simulink model "ThisOne-merged"  (R2026a)
settings: Solver=ode3  StopTime=2  FixedStep=1e-6  EnableMultiTasking=on
PreLoadFcn:
  | BLDCSpeedControlData;
values from neighbouring files (symbols this model uses):
  Jm = 4.97    [BLDCSpeedControlDataNewParam.m]
  p = 4    [BLDCSpeedControlDataNewParam.m]
undefined symbols (not defined in the file or in its folder): Ct_CqToRPM, Down, Up
libraries: nesl_utility x13, fl_lib x9, ee_lib x5, eeGeneralControl x2, eeBldcCurrentController x1, batt_lib x1, slpidlib x1, SignalEditorBlockLib x1
(part 1 of 2)
CloseFcn:
  | try,close(h1_BLDCSpeedControl),end
  | clear h1_BLDCSpeedControl
  | 
  | clear simlog_BLDCSpeedControl
  | clear logsout_BLDCSpeedControl
Description:
  | BLDC Speed Control
settings Model: PauseTimes=0.45  NumberOfSteps=10  Creator=The MathWorks, Inc.
settings DataIOCC: MaxDataPoints=210000  SignalLoggingName=logsout_BLDCSpeedControl
settings SimscapeCC: SimscapeNormalizeSystem=off  SimscapeNominalValues="[{\"value\":\"1\",\"unit\":\"A\"},{\"value\":\"1\",\"unit\":\"bar\"},{\"value\":\"1\",\"unit\":\"cm^2\"},{\"value\":\"1\",\"unit\":\"cm^3/s\"},{\"value\":\"1\",\"unit\":\"kJ/kg\"},{\"value\":\"1\",\"unit\":\"kW\"},{\"value\":\"1\",\"unit\":\"l\"},{\"value\":\"1\",\"unit\":\"N\"},{\"value\":\"1\",\"unit\":\"N*m\"},{\"value\":\"1\",\"unit\":\"V\"}]"  SimscapeLogSimulationStatistics=on  SimscapeLogName=simlog_BLDCSpeedControl  SimscapeLogLimitData=off  SimscapeLogDataHistory=210000.0

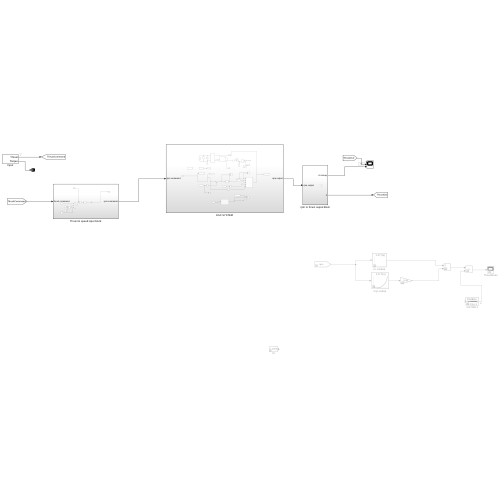
[thumbnail: Simulink's stored preview of the top-level diagram]
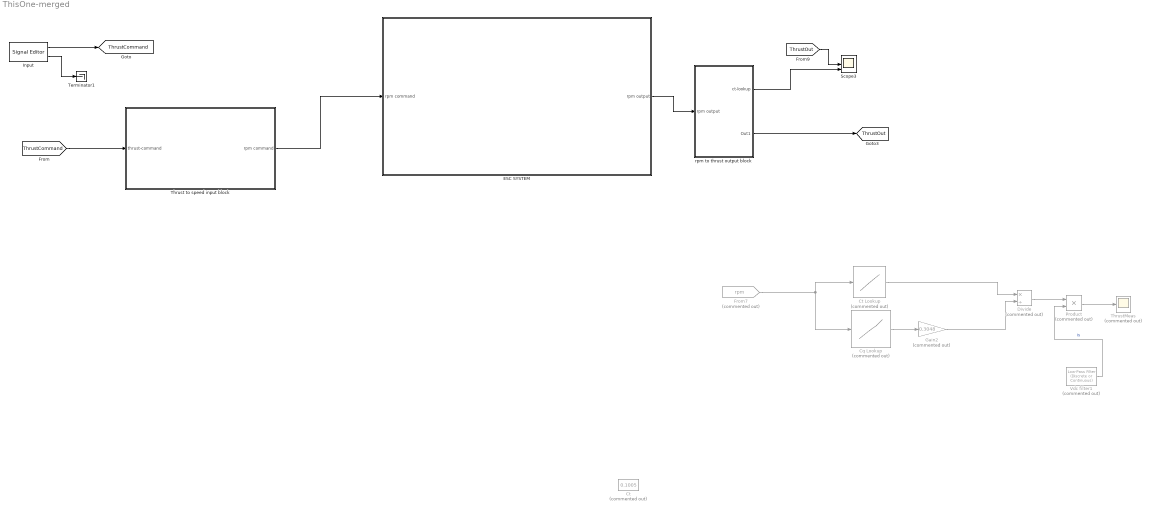
== system ThisOne-merged ==
  Cq Lookup : Lookup_n-D  Commented=on  NumberOfTableDimensions=1  BreakpointsForDimension1=Ct_CqToRPM.RPM  Table=Ct_CqToRPM.Cq  InternalRulePriority=Speed  RndMeth=Simplest
  Ct : Constant  Commented=on  Value=0.1005
  Ct Lookup : Lookup_n-D  Commented=on  NumberOfTableDimensions=1  BreakpointsForDimension1=Ct_CqToRPM.RPM  Table=Ct_CqToRPM.Ct  InternalRulePriority=Speed  RndMeth=Simplest
  Divide : Product  Commented=on  Inputs=*/
  ESC SYSTEM : Subsystem
  From7 : From  Commented=on  GotoTag=rpm  TagVisibility=global
  Gain2 : Gain  Commented=on  Gain=0.3048
  Input : SignalEditorBlockLib/Signal Editor  FileName=BLDCSpeedControlInput.mat  ActiveScenario=Test_1  ActiveSignal=Torque  IsBus=off  OutputBusObjectStr=Bus: BusObject  SampleTime=0  OutputAfterFinalValue=Extrapolation  Unit=inherit  PreserveSignalName=on  ApplySigPropsToAllScenarios=on  ApplySigPropsToAllSignals=off  SignalPropertySource=Dialog parameters
  Product : Product  Commented=on
  Scope3 : Scope  NumInputPorts=3
      settings: ActiveDisplayYMinimum=6.4992210204296432  ActiveDisplayYMaximum=7.577007831129519  DataLoggingVariableName=ScopeData11
  Terminator1 : Terminator
  Thrust to speed input block : Subsystem
  ThrustMeas : Scope  Commented=on
      settings: ActiveDisplayYMinimum=-0.61696410930468792  ActiveDisplayYMaximum=-0.5584126706390744  DataLoggingVariableName=ScopeData2
  Vdc filter1 : eeGeneralControl/Low-Pass Filter (Discrete or Continuous)  Commented=on  K=1  T=0.01  B=inf  A=-inf  init_option=Inherited from block input  x0=0  Ts=-1
  rpm to thrust output block : Subsystem
  tag scope: ThrustCommand=global, ThrustOut=global
  wires:
  Input/2 -> Terminator1/1
  Divide/1 -> Product/1
  Product/1 -> ThrustMeas/1
  Vdc filter1/1 -> Product/2  "is"
  From7/1 -> Cq Lookup/1, Ct Lookup/1
  Ct Lookup/1 -> Divide/1
  Gain2/1 -> Divide/2
  Cq Lookup/1 -> Gain2/1
  [ThrustOut] -> Scope3/2
  Thrust to speed input block/1(rpm command) -> ESC SYSTEM/1(rpm command)
  rpm to thrust output block/1(ct-lookup) -> Scope3/3
  rpm to thrust output block/2(Out1) -> [ThrustOut]
  Input/1 -> [ThrustCommand]
  [ThrustCommand] -> Thrust to speed input block/1(thrust-command)
  ESC SYSTEM/1(rpm output) -> rpm to thrust output block/1(rpm output)

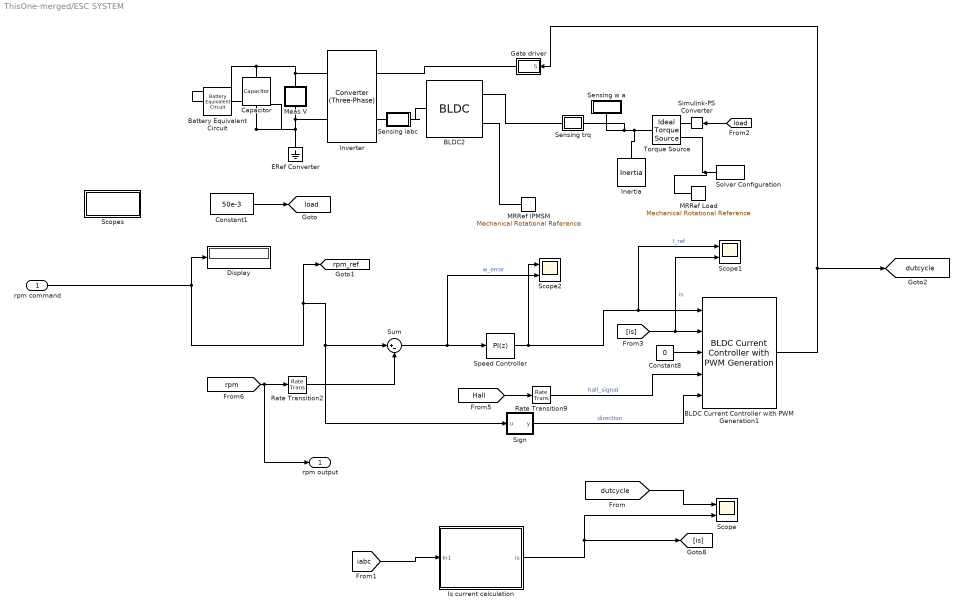
== system ThisOne-merged/ESC SYSTEM ==
  rpm command : Inport
  BLDC Current Controller with PWM Generation1 : eeBldcCurrentController/BLDC Current Controller with PWM Generation  Kp=0.5  Ki=10  Kaw=20  Ts=-1  Tsd=0.001  ActZC=off  CarrCount=Up-Down  Tper=1e-4  Tfundamental=Ts
      settings: LibrarySourceBlock=|
      | ee_sl_lib/BLDC Control/BLDC Current Controller
      | with PWM Generation
  BLDC2 : ee_lib/Electromechanical/Permanent Magnet/BLDC  port_option=ee.enum.threePhasePort.composite  rotor_param=ee.enum.pmsm.backemf.trapezoidflux  pm_flux_linkage=psim Wb  theta_constant=pi/(2*p) deg  emf_max=9.6 % Parameter not set V  w_meas=600 % Parameter not set rpm  DphiDtheta_tab=[0, -.1528, -.1528, .1528, .1528, 0] % Parameter not set Wb/rad  back_emf_tab=[0, -9.6, -9.6, 9.6, 9.6, 0] % Parameter not set V  rotor_angle_tab=[0, 7.5, 22.5, 37.5, 52.5, 60] % Parameter not set deg  nPolePairs=p  axes_param=ee.enum.rotorangle.qaxis  winding_type=ee.enum.electromech.statorconfiguration.wye  stator_param=ee.enum.statorparam.LdLqL0  machine_param=ee.enum.dqparameterization.constant  Ld=Ls H  Lq=Ls H  idVec=[-200, 0, 200] % Parameter not set A  iqVec=[-200, 0, 200] % Parameter not set A  LdMatrix=0.00022 * ones(3, 3) % Parameter not set H  LqMatrix=0.00022 * ones(3, 3) % Parameter not set H  L0=1.44 % Assumed inductance value mH  Ls=0.0002 % Parameter not set H  Lm=0 % Parameter not set H  Ms=0.00002 % Parameter not set H  Rs=Rs Ohm  zero_sequence=ee.enum.park.zerosequence.exclude  loss_param=ee.enum.ironloss.none  losses_oc=[0, 0, 0] % Parameter not set W  losses_sc=[0, 0, 0] % Parameter not set W  f_losses=60 % Parameter not set Hz  Isc_losses=95 % Parameter not set A  J=Jm cm^2*g  lam=Viscousfriction N*m*s/rad  i_d_specify=off  i_d_priority=None  i_d=0 A  i_d_nominal_specify=off  i_d_nominal_value=1  i_d_nominal_unit=A  i_q_specify=on  i_q_priority=None  i_q=0 A  i_q_nominal_specify=off  i_q_nominal_value=1  i_q_nominal_unit=A  torque_specify=on  torque_priority=None  torque=0 N*m  torque_nominal_specify=off  torque_nominal_value=1  torque_nominal_unit=N*m  angular_velocity_specify=off  angular_velocity_priority=High  angular_velocity=0 rpm  angular_velocity_nominal_specify=off  angular_velocity_nominal_value=1  angular_velocity_nominal_unit=rpm  angular_position_specify=off  angular_position_priority=High  angular_position=0 deg  angular_position_nominal_specify=off  angular_position_nominal_value=1  angular_position_nominal_unit=deg  alpha=3.93e-3 % Parameter not set 1/K  alpha_flux=-0.001 % Parameter not set 1/K  Tmeas=298.15 % Parameter not set K  stator_thermal_mass=100 % Parameter not set J/K  rotor_thermal_mass=200 % Parameter not set J/K  Rm_percent_rotor=90 % Parameter not set  Rd_percent_rotor=30 % Parameter not set  temperatureA_specify=off  temperatureA_priority=High  temperatureA=25 degC  temperatureA_nominal_specify=off  temperatureA_nominal_value=1  temperatureA_nominal_unit=degC  temperatureB_specify=off  temperatureB_priority=High  temperatureB=25 degC  temperatureB_nominal_specify=off  temperatureB_nominal_value=1  temperatureB_nominal_unit=degC  temperatureC_specify=off  temperatureC_priority=High  temperatureC=25 degC  temperatureC_nominal_specify=off  temperatureC_nominal_value=1  temperatureC_nominal_unit=degC  temperatureR_specify=off  temperatureR_priority=High  temperatureR=25 degC  temperatureR_nominal_specify=off  temperatureR_nominal_value=1  temperatureR_nominal_unit=degC
  Battery Equivalent Circuit : batt_lib/Cells/Battery Equivalent Circuit  PartSpecification="{\"CollectionId\":\"MW.SimscapeBattery\",\"CollectionVersion\":\"1.0.0\",\"DatasetId\":\"Molicel|INR_21700_P45B|simscape.battery.batteryEquivalentCircuit\",\"DisplayName\":\"Molicel:INR_21700_P45B\"}"  BatteryCapacity="4.493  hr*A"  ThermalModel=simscape.battery.enum.cells.BatteryThermalModel.ConstantTemperature  ExtrapolationMethod=simscape.enum.extrapolation.linear  SOCBreakpoints=[0 0.01 0.02 0.03 0.04 0.05 0.06 0.07 0.08 0.09 0.1 0.11 0.12 0.13 0.14 0.15 0.16 0.17 0.18 0.19 0.2 0.21 0.22 0.23 0.24 0.25 0.26 0.27 0.28 0.29 0.3 0.31 0.32 0.33 0.34 0.35 0.36 0.37 0.38 0.39 0.4 0.41 0.42 0.43 0.44 0.45 0.46 0.47 0.48 0.49 0.5 0.51 0.52 0.53 0.54 0.55 0.56 0.57 0.58 0.59 0.6 0.61 0.62 0.63 0.64 0.65 0.66 0.67 0.68 0.69 0.7 0.71 0.72 0.73 0.74 0.75 0.76 0.77 0.78 0.79 0.8 0.81 0.82 0.83 0.84 0.85 0.86 0.87 0.88 0.89 0.9 0.91 0.92 0.93 0.94 0.95 0.96 0.97 0.98 0.99 1] % Datasheet derived  TemperatureBreakpoints=[-40 -30 -20 0 23 45 60] % Datasheet derived degC  OpenCircuitVoltage=[3.17242 3.18272 3.19302 3.20331 3.21361 3.22391 3.23421 3.24451 3.25481 3.2651 3.2754 3.2857 3.296 3.3063 3.31659 3.32689 3.33719 3.34749 3.35779 3.36809 3.37838 3.38868 3.39898 3.40928 3.41958 3.42988 3.44017 3.45047 3.46077 3.47107 3.48137 3.49166 3.50196 3.51226 3.52256 3.53286 3.54316 3.55345 3.56375 3.57405 3.58435 3.59465 3.60495 3.61524 3.62554 3.63584 3.64614 3.65644 3.66673 3.67703 3.68733 3.69763 3.71041 3.72113 3.72997 3.73882 3.74912 3.75936 3.76951 3.7791 3.78865 3.79787 3.80709 3.8161 3.82509 3.83409 3.84308 3.85207 3.86107 3.87006 3.87901 3.88831 3.89824 3.90887 3.91951 3.93012 3.94073 3.95138 3.96184 3.97226 3.98268 3.99311 4.0032 4.01221 4.01944 4.02668 4.03286 4.03874 4.04383 4.0488 4.05377 4.05873 4.06312 4.06753 4.07333 4.08117 4.08904 4.09911 4.11111 4.13802 4.16831] % Datasheet derived V  OpenCircuitVoltageThermal="[3.17242 3.17242 3.17242 3.17242 3.17242 3.17242 3.17242;3.18272 3.18272 3.18272 3.18272 3.18272 3.18272 3.18272;3.19302 3.19302 3.19302 3.19302 3.19302 3.19302 3.19302;3.20331 3.20331 3.20331 3.20331 3.20331 3.20331 3.20331;3.21361 3.21361 3.21361 3.21361 3.21361 3.21361 3.21361;3.22391 3.22391 3.22391 3.22391 3.22391 3.22391 3.22391;3.23421 3.23421 3.23421 3.23421 3.23421 3.23421 3.23421;3.24451 3.24451 3.24451 3.24451 3.24451 3.24451 3.24451;3.25481 3.25481 3.25481 3.25481 3.25481 3.25481 3.25481;3.2651 3.2651 3.2651 3.2651 3.2651 3.2651 3.2651;3.2754 3.2754 3.2754 3.2754 3.2754 3.2754 3.2754;3.2857 3.2857 3.2857 3.2857 3.2857 3.2857 3.2857;3.296 3.296 3.296 3.296 3.296 3.296 3.296;3.3063 3.3063 3.3063 3.3063 3.3063 3.3063 3.3063;3.31659 3.31659 3.31659 3.31659 3.31659 3.31659 3.31659;3.32689 3.32689 3.32689 3.32689 3.32689 3.32689 3.32689;3.33719 3.33719 3.33719 3.33719 3.33719 3.33719 3.33719;3.34749 3.34749 3.34749 3.34749 3.34749 3.34749 3.34749;3.35779 3.35779 3.35779 3.35779 3.35779 3.35779 3.35779;3.36809 3.36809 3.36809 3.36809 3.36809 3.36809 3.36809;3.37838 3.37838 3.37838 3.37838 3.37838 3.37838 3.37838;3.38868 3.38868 3.38868 3.38868 3.38868 3.38868 3.38868;3.39898 3.39898 3.39898 3.39898 3.39898 3.39898 3.39898;3.40928 3.40928 3.40928 3.40928 3.40928 3.40928 3.40928;3.41958 3.41958 3.41958 3.41958 3.41958 3.41958 3.41958;3.42988 3.42988 3.42988 3.42988 3.42988 3.42988 3.42988;3.44017 3.44017 3.44017 3.44017 3.44017 3.44017 3.44017;3.45047 3.45047 3.45047 3.45047 3.45047 3.45047 3.45047;3.46077 3.46077 3.46077 3.46077 3.46077 3.46077 3.46077;3.47107 3.47107 3.47107 3.47107 3.47107 3.47107 3.47107;3.48137 3.48137 3.48137 3.48137 3.48137 3.48137 3.48137;3.49166 3.49166 3.49166 3.49166 3.49166 3.49166 3.49166;3.50196 3.50196 3.50196 3.50196 3.50196 3.50196 3.50196;3.51226 3.51226 3.51226 3.51226 3.51226 3.51226 3.51226;3.52256 3.52256 3.52256 3.52256 3.52256 3.52256 3.52256;3.53286 3.53286 3.53286 3.53286 3.53286 3.53286 3.53286;3.54316 3.54316 3.54316 3.54316 3.54316 3.54316 3.54316;3.55345 3.55345 3.55345 3.55345 3.55345 3.55345 3.55345;3.56375 3.56375 3.56375 3.56375 3.56375 3.56375 3.56375;3.57405 3.57405 3.57405 3.57405 3.57405 3.57405 3.57405;3.58435 3.58435 3.58435 3.58435 3.58435 3.58435 3.58435;3.59465 3.59465 3.59465 3.59465 3.59465 3.59465 3.59465;3.60495 3.60495 3.60495 3.60495 3.60495 3.60495 3.60495;3.61524 3.61524 3.61524 3.61524 3.61524 3.61524 3.61524;3.62554 3.62554 3.62554 3.62554 3.62554 3.62554 3.62554;3.63584 3.63584 3.63584 3.63584 3.63584 3.63584 3.63584;3.64614 3.64614 3.64614 3.64614 3.64614 3.64614 3.64614;3.65644 3.65644 3.65644 3.65644 3.65644 3.65644 3.65644;3.66673 3.66673 3.66673 3.66673 3.66673 3.66673 3.66673;3.67703 3.67703 3.67703 3.67703 3.67703 3.67703 3.67703;3.68733 3.68733 3.68733 3.68733 3.68733 3.68733 3.68733;3.69763 3.69763 3.69763 3.69763 3.69763 3.69763 3.69763;3.71041 3.71041 3.71041 3.71041 3.71041 3.71041 3.71041;3.72113 3.72113 3.72113 3.72113 3.72113 3.72113 3.72113;3.72997 3.72997 3.72997 3.72997 3.72997 3.72997 3.72997;3.73882 3.73882 3.73882 3.73882 3.73882 3.73882 3.73882;3.74912 3.74912 3.74912 3.74912 3.74912 3.74912 3.74912;3.75936 3.75936 3.75936 3.75936 3.75936 3.75936 3.75936;3.76951 3.76951 3.76951 3.76951 3.76951 3.76951 3.76951;3.7791 3.7791 3.7791 3.7791 3.7791 3.7791 3.7791;3.78865 3.78865 3.78865 3.78865 3.78865 3.78865 3.78865;3.79787 3.79787 3.79787 3.79787 3.79787 3.79787 3.79787;3.80709 3.80709 3.80709 3.80709 3.80709 3.80709 3.80709;3.8161 3.8161 3.8161 3.8161 3.8161 3.8161 3.8161;3.82509 3.82509 3.82509 3.82509 3.82509 3.82509 3.82509;3.83409 3.83409 3.83409 3.83409 3.83409 3.83409 3.83409;3.84308 3.84308 3.84308 3.84308 3.84308 3.84308 3.84308;3.85207 3.85207 3.85207 3.85207 3.85207 3.85207 3.85207;3.86107 3.86107 3.86107 3.86107 3.86107 3.86107 3.86107;3.87006 3.87006 3.87006 3.87006 3.87006 3.87006 3.87006;3.87901 3.87901 3.87901 3.87901 3.87901 3.87901 3.87901;3.88831 3.88831 3.88831 3.88831 3.88831 3.88831 3.88831;3.89824 3.89824 ...(+1594 chars)] *12  V"  VoltageRange=[3.4 Inf] *12 V  HysteresisModel=simscape.battery.enum.cells.HysteresisModel.none  MaximumHysteresisVoltage=[0, 0, 0, 0, 0, 0, 0] % Parameter not set V  InstantaneousHysteresisVoltage=[0, 0, 0, 0, 0, 0, 0] % Parameter not set V  HysteresisRate=0.1 % Parameter not set  MaximumHysteresisVoltageThermal=[0, 0, 0; 0, 0, 0; 0, 0, 0; 0, 0, 0; 0, 0, 0; 0, 0, 0; 0, 0, 0] % Parameter not set V  InstantaneousHysteresisVoltageThermal=[0, 0, 0; 0, 0, 0; 0, 0, 0; 0, 0, 0; 0, 0, 0; 0, 0, 0; 0, 0, 0] % Parameter not set V  HysteresisRateThermal=0.1 % Parameter not set  ResistanceSOCBreakpoints=[0 0.01 0.02 0.03 0.04 0.05 0.06 0.07 0.08 0.09 0.1 0.11 0.12 0.13 0.14 0.15 0.16 0.17 0.18 0.19 0.2 0.21 0.22 0.23 0.24 0.25 0.26 0.27 0.28 0.29 0.3 0.31 0.32 0.33 0.34 0.35 0.36 0.37 0.38 0.39 0.4 0.41 0.42 0.43 0.44 0.45 0.46 0.47 0.48 0.49 0.5 0.51 0.52 0.53 0.54 0.55 0.56 0.57 0.58 0.59 0.6 0.61 0.62 0.63 0.64 0.65 0.66 0.67 0.68 0.69 0.7 0.71 0.72 0.73 0.74 0.75 0.76 0.77 0.78 0.79 0.8 0.81 0.82 0.83 0.84 0.85 0.86 0.87 0.88 0.89 0.9 0.91 0.92 0.93 0.94 0.95 0.96 0.97 0.98 0.99 1] % Datasheet derived  ResistanceTemperatureBreakpoints="[-40 -30 -20 0 23 45 60]  degC"  ResistanceCurrentBreakpoints=[-1, 0, 1] % Parameter not set A  CurrentDependence=simscape.battery.enum.cells.CurrentDependence.Disabled  R0=[0.02095 0.01921 0.01774 0.0166 0.01557 0.01469 0.01398 0.01338 0.01283 0.01239 0.01196 0.01155 0.01116 0.01079 0.01042 0.01007 0.00974 0.00949 0.00924 0.009 0.00876 0.00855 0.00843 0.00832 0.00826 0.00825 0.00825 0.00826 0.00827 0.00828 0.0083 0.00834 0.00838 0.00842 0.00848 0.00855 0.00863 0.00871 0.00879 0.00887 0.00895 0.00903 0.00911 0.00918 0.00925 0.00931 0.00938 0.00946 0.00953 0.00961 0.00968 0.00976 0.00991 0.01 0.01003 0.01006 0.01013 0.01022 0.0103 0.01037 0.01043 0.01049 0.01055 0.01061 0.01066 0.01072 0.01077 0.01082 0.01088 0.01093 0.01099 0.01105 0.01114 0.01125 0.01136 0.01148 0.01161 0.01175 0.01188 0.01202 0.01215 0.01228 0.01241 0.01253 0.01261 0.01269 0.01275 0.0128 0.01285 0.01289 0.01294 0.01298 0.01296 0.01292 0.01292 0.01288 0.01282 0.0128 0.01232 0.01214 0.00952] % Datasheet derived Ohm  R0I=[.0117, .0085, .009; .011, .0085, .009; .0114, .0087, .0092; .0107, .0082, .0088; .0107, .0083, .0091; .0113, .0085, .0089; .0116, .0085, .0089] % Parameter not set Ohm  R0Thermal=[0.3026 0.35142 0.34349 0.24415 0.02095 0.15874 0.14729;0.2941 0.33555 0.32379 0.22614 0.01921 0.13363 0.12249;0.28559 0.31969 0.30408 0.20813 0.01774 0.10853 0.10276;0.27709 0.30382 0.28438 0.19012 0.0166 0.09423 0.0861;0.26858 0.28796 0.26468 0.17211 0.01557 0.07998 0.0748;0.26008 0.27209 0.24498 0.1541 0.01469 0.07024 0.06679;0.25157 0.25623 0.22527 0.1361 0.01398 0.06387 0.05877;0.24307 0.24036 0.20557 0.11861 0.01338 0.0575 0.05275;0.23456 0.2245 0.18587 0.10674 0.01283 0.05113 0.04899;0.22606 0.20863 0.16617 0.09525 0.01239 0.04679 0.04522;0.21755 0.19277 0.14651 0.08799 0.01196 0.0439 0.04145;0.20905 0.1769 0.13098 0.08073 0.01155 0.04101 0.03817;0.20054 0.16103 0.11905 0.07347 0.01116 0.03813 0.03522;0.19204 0.14769 0.11102 0.06895 0.01079 0.03524 0.03228;0.18353 0.13913 0.10517 0.06499 0.01042 0.03235 0.02934;0.17503 0.13157 0.09933 0.06104 0.01007 0.02946 0.0264;0.16653 0.1271 0.09371 0.05708 0.00974 0.02657 0.02345;0.15804 0.12264 0.09094 0.05312 0.00949 0.02417 0.02125;0.15354 0.11817 0.08816 0.04917 0.00924 0.02286 0.01972;0.14976 0.11385 0.08539 0.04748 0.009 0.02156 0.0182;0.14598 0.11213 0.08261 0.04617 0.00876 0.02025 0.01667;0.14219 0.11042 0.08103 0.04487 0.00855 0.01894 0.01515;0.14033 0.10871 0.08035 0.04356 0.00843 0.01763 0.01363;0.13876 0.10699 0.07967 0.04225 0.00832 0.01632 0.0121;0.13718 0.10528 0.07899 0.04094 0.00826 0.01501 0.01058;0.13561 0.10357 0.07831 0.03964 0.00825 0.0137 0.00906;0.13404 0.10198 0.07763 0.03833 0.00825 0.01239 0.00753;0.13247 0.10119 0.07695 0.03702 0.00826 0.01108 0.0065;0.13096 0.10039 0.07627 0.03624 0.00827 0.00977 0.00633;0.13043 0.0996 0.07559 0.03615 0.00828 0.00846 0.00617;0.1299 0.0988 0.07491 0.03606 0.0083 0.00774 0.006;0.12937 0.09801 0.07423 0.03597 0.00834 0.00779 0.00583;0.12883 0.09721 0.07355 0.03588 0.00838 0.00783 0.00567;0.1283 0.09642 0.07301 0.03579 0.00842 0.00787 0.0055;0.12777 0.09585 0.07296 0.0357 0.00848 0.00792 0.00534;0.12724 0.09584 0.07291 0.03561 0.00855 0.00796 0.00517;0.12675 0.09584 0.07286 0.03552 0.00863 0.00801 0.005;0.12643 0.09583 0.0728 0.03543 0.00871 0.00805 0.00484;0.12611 0.09582 0.07275 0.03534 0.00879 0.00809 0.00467;0.12579 0.09582 0.0727 0.03525 0.00887 0.00814 0.0045;0.12547 0.09581 0.07264 0.03526 0.00895 0.00818 0.00434;0.12514 0.0958 0.07259 0.03537 0.00903 0.00823 0.00405;0.12482 0.09579 0.07254 0.03547 0.00911 0.00804 0.00366;0.1245 0.09579 0.07248 0.03558 0.00918 0.00776 0.00327;0.12418 0.09578 0.07243 0.03568 0.00925 0.00748 0.00287;0.12386 0.09577 0.07231 0.03579 0.00931 0.0072 0.00248;0.12354 0.09576 0.0721 0.03589 0.00938 0.00692 0.00209;0.12322 0.09576 0.07189 0.036 0.00946 0.00664 0.0017;0.12301 0.09575 0.07168 0.03611 0.00953 0.00636 0.00131;0.12309 0.09574 0.07147 0.03621 0.00961 0.00608 0.00092;0.12318 0.09573 0.07125 0.0363 0.00968 0.0058 0.00053;0.12326 0.09573 0.07104 0.03637 0.00976 0.00552 0.00014;0.12389 0.09628 0.07138 0.03699 0.00991 0.00579 0.0003;0.12407 0.09637 0.07126 0.03715 0.01 0.0056 0.0003;0.12383 0.09605 0.07073 0.0369 0.01003 0.00504 0.0003;0.12359 0.09573 0.07019 0.03664 0.01006 0.00503 0.0003;0.12367 0.09573 0.06998 0.03671 0.01013 0.00534 0.00063;0.12375 0.09572 0.06975 0.03677 0.01022 0.00564 0.00094;0.1238 0.09569 0.07006 0.0368 0.0103 0.00593 0.00123;0.12372 0.09554 0.07026 0.03671 0.01037 0.00608 0.00139;0.12364 0.09537 0.07046 0.03661 0.01043 0.00623 0.00155;0.12348 0.09514 0.07058 0.03644 0.01049 0.0063 0.00163;0.12333 0.0949 0.07071 0.03627 0.01055 0.00638 0.00171;0.12312 0.09461 0.07078 0.03605 0.01061 0.00641 0.00175;0.12291 0.09433 0.07085 0.03583 0.01066 0.00643 0.00168;0.12271 0.09404 0.07093 0.03568 0.01072 0.00646 0.00161;0.12275 0.09398 0.071 0.03622 0.01077 0.00646 0.00153;0.12316 0.09449 0.07107 0.03677 0.01082 0.00636 0.00145;0.12357 0.095 0.07115 0.03731 0.01088 0.00625 0.00137;0.12398 0.09551 0.07151 0.03785 0.01093 0.00614 0.00129;0.12438 0.09601 0.07221 0.03839 0.01099 0.00602 0.0012;0.12486 0.09659 0.07299 0.039 0.01105 0.00599 0.00119;0.12548 0.09731 0.07391 ...(+1579 chars)] % Datasheet derived Ohm  R0ThermalI=repmat([.0117, .0085, .009; .011, .0085, .009; .0114, .0087, .0092; .0107, .0082, .0088; .0107, .0083, .0091; .0113, .0085, .0089; .0116, .0085, .0089], 1, 1, 3) % Parameter not set Ohm  DischargeR0=[.0085, .0085, .0087, .0082, .0083, .0085, .0085] % Parameter not set Ohm  ChargeR0=[.0085, .0085, .0087, .0082, .0083, .0085, .0085] % Parameter not set Ohm  ChargeR0Thermal=[.0117, .0085, .009; .011, .0085, .009; .0114, .0087, .0092; .0107, .0082, .0088; .0107, .0083, .0091; .0113, .0085, .0089; .0116, .0085, .0089] % Parameter not set Ohm  DischargeR0Thermal=[.0117, .0085, .009; .011, .0085, .009; .0114, .0087, .0092; .0107, .0082, .0088; .0107, .0083, .0091; .0113, .0085, .0089; .0116, .0085, .0089] % Parameter not set Ohm  RCPairs=simscape.battery.enum.cells.RCPairs.noDynamics  R1=[.0029, .0024, .0026, .0016, .0023, .0018, .0017] % Parameter not set Ohm  Tau1=[36, 45, 105, 29, 77, 33, 39] % Parameter not set s  R2=[.0029, .0024, .0026, .0016, .0023, .0018, .0017] % Parameter not set Ohm  Tau2=[36, 45, 105, 29, 77, 33, 39] % Parameter not set s  R3=[.0029, .0024, .0026, .0016, .0023, .0018, .0017] % Parameter not set Ohm  Tau3=[36, 45, 105, 29, 77, 33, 39] % Parameter not set s  R1I=[.0109, .0029, .0013; .0069, .0024, .0012; .0047, .0026, .0013; .0034, .0016, .001; .0033, .0023, .0014; .0033, .0018, .0011; .0028, .0017, .0011] % Parameter not set Ohm  Tau1I=[20, 36, 39; 31, 45, 39; 109, 105, 61; 36, 29, 26; 59, 77, 67; 40, 33, 29; 25, 39, 33] % Parameter not set s  R2I=[.0109, .0029, .0013; .0069, .0024, .0012; .0047, .0026, .0013; .0034, .0016, .001; .0033, .0023, .0014; .0033, .0018, .0011; .0028, .0017, .0011] % Parameter not set Ohm  Tau2I=[20, 36, 39; 31, 45, 39; 109, 105, 61; 36, 29, 26; 59, 77, 67; 40, 33, 29; 25, 39, 33] % Parameter not set s  R3I=[.0109, .0029, .0013; .0069, .0024, .0012; .0047, .0026, .0013; .0034, .0016, .001; .0033, .0023, .0014; .0033, .0018, .0011; .0028, .0017, .0011] % Parameter not set Ohm  Tau3I=[20, 36, 39; 31, 45, 39; 109, 105, 61; 36, 29, 26; 59, 77, 67; 40, 33, 29; 25, 39, 33] % Parameter not set s  DischargeR1=[.0029, .0024, .0026, .0016, .0023, .0018, .0017] % Parameter not set Ohm  DischargeTau1=[36, 45, 105, 29, 77, 33, 39] % Parameter not set s  ChargeR1=[.0029, .0024, .0026, .0016, .0023, .0018, .0017] % Parameter not set Ohm  ChargeTau1=[36, 45, 105, 29, 77, 33, 39] % Parameter not set s  DischargeR2=[.0029, .0024, .0026, .0016, .0023, .0018, .0017] % Parameter not set Ohm  DischargeTau2=[36, 45, 105, 29, 77, 33, 39] % Parameter not set s  ChargeR2=[.0029, .0024, .0026, .0016, .0023, .0018, .0017] % Parameter not set Ohm  ChargeTau2=[36, 45, 105, 29, 77, 33, 39] % Parameter not set s  DischargeR3=[.0029, .0024, .0026, .0016, .0023, .0018, .0017] % Parameter not set Ohm  DischargeTau3=[36, 45, 105, 29, 77, 33, 39] % Parameter not set s  ChargeR3=[.0029, .0024, .0026, .0016, .0023, .0018, .0017] % Parameter not set Ohm  ChargeTau3=[36, 45, 105, 29, 77, 33, 39] % Parameter not set s  R1Thermal=[.0109, .0029, .0013; .0069, .0024, .0012; .0047, .0026, .0013; .0034, .0016, .001; .0033, .0023, .0014; .0033, .0018, .0011; .0028, .0017, .0011] % Parameter not set Ohm  Tau1Thermal=[20, 36, 39; 31, 45, 39; 109, 105, 61; 36, 29, 26; 59, 77, 67; 40, 33, 29; 25, 39, 33] % Parameter not set s  R2Thermal=[.0109, .0029, .0013; .0069, .0024, .0012; .0047, .0026, .0013; .0034, .0016, .001; .0033, .0023, .0014; .0033, .0018, .0011; .0028, .0017, .0011] % Parameter not set Ohm  Tau2Thermal=[20, 36, 39; 31, 45, 39; 109, 105, 61; 36, 29, 26; 59, 77, 67; 40, 33, 29; 25, 39, 33] % Parameter not set s  R3Thermal=[.0109, .0029, .0013; .0069, .0024, .0012; .0047, .0026, .0013; .0034, .0016, .001; .0033, .0023, .0014; .0033, .0018, .0011; .0028, .0017, .0011] % Parameter not set Ohm  Tau3Thermal=[20, 36, 39; 31, 45, 39; 109, 105, 61; 36, 29, 26; 59, 77, 67; 40, 33, 29; 25, 39, 33] % Parameter not set s  R1ThermalI=repmat([.0109, .0029, .0013; .0069, .0024, .0012; .0047, .0026, .0013; .0034, .0016, .001; .0033, .0023, .0014; .0033, .0018, .0011; .0028, .0017, .0011], 1, 1, 3) % Parameter not set Ohm  Tau1ThermalI=repmat([20, 36, 39; 31, 45, 39; 109, 105, 61; 36, 29, 26; 59, 77, 67; 40, 33, 29; 25, 39, 33], 1, 1, 3) % Parameter not set s  R2ThermalI=repmat([.0109, .0029, .0013; .0069, .0024, .0012; .0047, .0026, .0013; .0034, .0016, .001; .0033, .0023, .0014; .0033, .0018, .0011; .0028, .0017, .0011], 1, 1, 3) % Parameter not set Ohm  Tau2ThermalI=repmat([20, 36, 39; 31, 45, 39; 109, 105, 61; 36, 29, 26; 59, 77, 67; 40, 33, 29; 25, 39, 33], 1, 1, 3) % Parameter not set s  R3ThermalI=repmat([.0109, .0029, .0013; .0069, .0024, .0012; .0047, .0026, .0013; .0034, .0016, .001; .0033, .0023, .0014; .0033, .0018, .0011; .0028, .0017, .0011], 1, 1, 3) % Parameter not set Ohm  Tau3ThermalI=repmat([20, 36, 39; 31, 45, 39; 109, 105, 61; 36, 29, 26; 59, 77, 67; 40, 33, 29; 25, 39, 33], 1, 1, 3) % Parameter not set s  DischargeR1Thermal=[.0109, .0029, .0013; .0069, .0024, .0012; .0047, .0026, .0013; .0034, .0016, .001; .0033, .0023, .0014; .0033, .0018, .0011; .0028, .0017, .0011] % Parameter not set Ohm  DischargeTau1Thermal=[20, 36, 39; 31, 45, 39; 109, 105, 61; 36, 29, 26; 59, 77, 67; 40, 33, 29; 25, 39, 33] % Parameter not set s  ChargeR1Thermal=[.0109, .0029, .0013; .0069, .0024, .0012; .0047, .0026, .0013; .0034, .0016, .001; .0033, .0023, .0014; .0033, .0018, .0011; .0028, .0017, .0011] % Parameter not set Ohm  ChargeTau1Thermal=[20, 36, 39; 31, 45, 39; 109, 105, 61; 36, 29, 26; 59, 77, 67; 40, 33, 29; 25, 39, 33] % Parameter not set s  DischargeR2Thermal=[.0109, .0029, .0013; .0069, .0024, .0012; .0047, .0026, .0013; .0034, .0016, .001; .0033, .0023, .0014; .0033, .0018, .0011; .0028, .0017, .0011] % Parameter not set Ohm  DischargeTau2Thermal=[20, 36, 39; 31, 45, 39; 109, 105, 61; 36, 29, 26; 59, 77, 67; 40, 33, 29; 25, 39, 33] % Parameter not set s  ChargeR2Thermal=[.0109, .0029, .0013; .0069, .0024, .0012; .0047, .0026, .0013; .0034, .0016, .001; .0033, .0023, .0014; .0033, .0018, .0011; .0028, .0017, .0011] % Parameter not set Ohm  ChargeTau2Thermal=[20, 36, 39; 31, 45, 39; 109, 105, 61; 36, 29, 26; 59, 77, 67; 40, 33, 29; 25, 39, 33] % Parameter not set s  DischargeR3Thermal=[.0109, .0029, .0013; .0069, .0024, .0012; .0047, .0026, .0013; .0034, .0016, .001; .0033, .0023, .0014; .0033, .0018, .0011; .0028, .0017, .0011] % Parameter not set Ohm  DischargeTau3Thermal=[20, 36, 39; 31, 45, 39; 109, 105, 61; 36, 29, 26; 59, 77, 67; 40, 33, 29; 25, 39, 33] % Parameter not set s  ChargeR3Thermal=[.0109, .0029, .0013; .0069, .0024, .0012; .0047, .0026, .0013; .0034, .0016, .001; .0033, .0023, .0014; .0033, .0018, .0011; .0028, .0017, .0011] % Parameter not set Ohm  ChargeTau3Thermal=[20, 36, 39; 31, 45, 39; 109, 105, 61; 36, 29, 26; 59, 77, 67; 40, 33, 29; 25, 39, 33] % Parameter not set s  SelfDischargeResistor=simscape.battery.enum.cells.BatteryEnable.Disabled  SelfDischargeR=7e3 % Parameter not set Ohm  SelfDischargeRThermal=[8000, 7000, 6000] % Parameter not set Ohm  CyclingAgingMethod=simscape.battery.enum.cells.CyclingAgingMethod.tableN  CycleCalculationMethod=simscape.battery.enum.cells.CycleCalculationMethod.EquivalentCycles  NumDisCycles=100 % Parameter not set  OCVChange=0 % Parameter not set  R0Change=0 % Parameter not set  CapacityChange=0 % Parameter not set  SelfDischargeRChange=0 % Parameter not set  R1Change=0 % Parameter not set  R2Change=0 % Parameter not set  R3Change=0 % Parameter not set  NumDisCyclesBreakpoints=[0 6 11 16 21 26 31 36 41 46 51 56 61 66 71 76 81 86 91 96 101 106 111 116 121 126 131 136 141 146 151 156 161 166 171 176 181 186 191 196 201 206 211 216 221 226 231 236 241 246 251 256 261 266 271 276 281 286 291 296 301 306 311 316 321 326 331 336 341 346 351 356 361 366 371 376 381 386 391 396 401 406 411 416 421 426 431 436 441 446 451 456 461 466 471 476 481 486 491 496] % Datasheet derived  AgingTemperatureBreakpoints=[298.15, 323.15] % Parameter not set K  AgingCurrentBreakpoints=[-.1, -.5, -5] % Parameter not set A  OCVChangeVec=[0 -0.0674 -0.1349 -0.2023 -0.2697 -0.3371 -0.4046 -0.472 -0.5394 -0.6069 -0.6828 -0.7561 -0.8245 -0.8929 -0.9613 -1.0297 -1.0981 -1.1664 -1.2348 -1.3032 -1.3773 -1.4186 -1.4598 -1.5011 -1.5424 -1.5836 -1.6249 -1.6652 -1.6999 -1.7345 -1.7691 -1.8038 -1.8384 -1.8731 -1.908 -1.9398 -1.9715 -2.0033 -2.0351 -2.0669 -2.0986 -2.1303 -2.162 -2.1976 -2.2332 -2.2687 -2.2977 -2.3239 -2.3502 -2.3765 -2.4028 -2.4264 -2.4464 -2.4663 -2.4863 -2.5063 -2.5263 -2.5462 -2.5661 -2.5849 -2.6031 -2.6212 -2.6407 -2.6612 -2.6817 -2.7022 -2.7227 -2.7432 -2.7637 -2.7842 -2.8047 -2.8253 -2.8458 -2.8662 -2.8858 -2.9054 -2.9249 -2.9445 -2.9641 -2.9837 -3.0037 -3.0238 -3.0439 -3.064 -3.0841 -3.1042 -3.1267 -3.1499 -3.1731 -3.1989 -3.2248 -3.2508 -3.2781 -3.3053 -3.3326 -3.3598 -3.387 -3.4171 -3.449 -3.4809] % Datasheet derived  OCVChangeThermal=[0, 0; 0, 0; 0, 0; 0, 0] % Parameter not set  R0ChangeVec=[0 0 0 0 0 0 0 0 0 0 0 0 0 0 0 0 0 0 0 0 0 0 0 0 0 0 0 0 0 0 0 0 0 0 0 0 0 0 0 0 0 0 0 0 0 0 0 0 0 0 0 0 0 0 0 0 0 0 0 0 0 0 0 0 0 0 0 0 0 0 0 0 0 0 0 0 0 0 0 0 0 0 0 0 0 0 0 0 0 0 0 0 0 0 0 0 0 0 0 0] % Parameter assumed  R0ChangeThermal=[0, 0; 0, 0; 0, 0; 0, 0] % Parameter not set  R0ChangeThermalI=repmat(0, 4, 2, 3) % Parameter not set  R0CyclingChangeInitialTarget=0 % Parameter not set  CapacityChangeVec=[0 -0.093 -0.186 -0.278 -0.371 -0.464 -0.557 -0.649 -0.742 -0.835 -0.94 -1.045 -1.151 -1.257 -1.363 -1.469 -1.575 -1.681 -1.787 -1.893 -2.017 -2.161 -2.304 -2.447 -2.591 -2.734 -2.877 -3.021 -3.164 -3.307 -3.451 -3.594 -3.737 -3.881 -4.032 -4.201 -4.369 -4.538 -4.706 -4.874 -5.043 -5.211 -5.38 -5.569 -5.758 -5.947 -6.135 -6.324 -6.513 -6.702 -6.891 -7.08 -7.269 -7.458 -7.647 -7.836 -8.025 -8.214 -8.403 -8.582 -8.754 -8.927 -9.099 -9.271 -9.443 -9.615 -9.787 -9.96 -10.132 -10.304 -10.476 -10.648 -10.82 -10.992 -11.156 -11.32 -11.485 -11.649 -11.814 -11.978 -12.143 -12.307 -12.471 -12.636 -12.8 -12.965 -13.129 -13.293 -13.458 -13.641 -13.825 -14.008 -14.192 -14.376 -14.56 -14.743 -14.927 -15.111 -15.295 -15.478] % Datasheet derived  CapacityChangeThermal=[0, 0; 0, 0; 0, 0; 0, 0] % Parameter not set  CapacityChangeThermalI=repmat(0, 4, 2, 3) % Parameter not set  CapacityCyclingChangeInitialTarget=0 % Parameter not set  SelfDischargeRChangeVec=[0, 0, 0, 0] % Parameter not set  SelfDischargeRChangeThermal=[0, 0; 0, 0; 0, 0; 0, 0] % Parameter not set  SelfDischargeRChangeThermalI=repmat(0, 4, 2, 3) % Parameter not set  SelfDischargeRCyclingChangeInitialTarget=0 % Parameter not set  R1ChangeVec=[0, 0, 0, 0] % Parameter not set  R1ChangeThermal=[0, 0; 0, 0; 0, 0; 0, 0] % Parameter not set  R1ChangeThermalI=repmat(0, 4, 2, 3) % Parameter not set  R1CyclingChangeInitialTarget=0 % Parameter not set  R2ChangeVec=[0, 0, 0, 0] % Parameter not set  R2ChangeThermal=[0, 0; 0, 0; 0, 0; 0, 0] % Parameter not set  R2ChangeThermalI=repmat(0, 4, 2, 3) % Parameter not set  R2CyclingChangeInitialTarget=0 % Parameter not set  R3ChangeVec=[0, 0, 0, 0] % Parameter not set  R3ChangeThermal=[0, 0; 0, 0; 0, 0; 0, 0] % Parameter not set  R3ChangeThermalI=repmat(0, 4, 2, 3) % Parameter not set  R3CyclingChangeInitialTarget=0 % Parameter not set  CalendarAgeResistance=simscape.battery.enum.cells.BatteryEnable.Disabled  CalendarAgeCapacity=simscape.battery.enum.cells.BatteryEnable.Disabled  CalendarAgingMethod=simscape.battery.enum.cells.CalendarAgingMethod.equation  StorageVariable=simscape.battery.enum.cells.StorageVariable.OCV  OCVDuringStorage=0.9 % Parameter not set  SOCDuringStorage=0.6 % Parameter not set  StorageTimeIntervals=[0] % Parameter not set d  StorageTemperatures=[273] % Parameter not set K  ResistanceScalingOCV=2.2134e6 % Parameter not set  ResistanceScalingOCVOffset=1.632e6 % Parameter not set  ResistanceExponentialIncrease=0.515833569 % Parameter not set V  ResistanceTimeExponent=0.75 % Parameter not set  ResistanceAgeTemperatureBreakpoints=[273.15, 298.15, 323.15] % Parameter not set K  ResistanceAgeTimeBreakpoints=[0, 90, 180, 270] % Parameter not set d  PercentResistanceChange=[0, 0, 0] % Parameter not set  ResistanceTimeBreakpoints=100 % Parameter not set d  PercentResistanceChangeThermal=[0, 0, 0; 0, 0, 0; 0, 0, 0; 0, 0, 0] % Parameter not set  CapacityScalingOCV=1.5097e07 % Parameter not set  CapacityScalingOCVOffset=8.3625e06 % Parameter not set  CapacityExponentialIncrease=0.6011 % Parameter not set V  CapacityTimeExponent=0.75 % Parameter not set  CapacityAgeTemperatureBreakpoints=[273.15, 298.15, 323.15] % Parameter not set K  CapacityAgeTimeBreakpoints=[0, 90, 180, 270] % Parameter not set d  PercentCapacityChange=[0, 0, 0] % Parameter not set  CapacityTimeBreakpoints=100 % Parameter not set d  PercentCapacityChangeThermal=[0, 0, 0; 0, 0, 0; 0, 0, 0; 0, 0, 0] % Parameter not set  SimulationTemperature=298.15 % Parameter not set K  BatteryThermalMass=63 % Parameter assumed J/K  NumThermalModels=6 % Parameter not set  ThermalConductivityZ=18 % Parameter not set W/(K*m)  CrossSectionalAreaXY=0.000365 m^2  Height=0.0702 m  ReversibleHeatModel=simscape.battery.enum.cells.ReversibleHeatModel.Disabled  EntropicCoefficient=[0, 0, 0, 0, 0, 0, 0] % Parameter not set mV/K  CurrentDirectionality=simscape.battery.enum.cells.BatteryEnable.Disabled  stateOfCharge_specify=off  stateOfCharge_priority=High  stateOfCharge=1  stateOfCharge_nominal_specify=off  stateOfCharge_nominal_value=1  stateOfCharge_nominal_unit=1  batteryVoltage_specify=off  batteryVoltage_priority=None  batteryVoltage=0 V  batteryVoltage_nominal_specify=off  batteryVoltage_nominal_value=1  batteryVoltage_nominal_unit=V  batteryCurrent_specify=off  batteryCurrent_priority=None  batteryCurrent=0 A  batteryCurrent_nominal_specify=off  batteryCurrent_nominal_value=1  batteryCurrent_nominal_unit=A  numCycles_specify=off  numCycles_priority=High  numCycles=0  numCycles_nominal_specify=off  numCycles_nominal_value=1  numCycles_nominal_unit=1  batteryTemperature_specify=off  batteryTemperature_priority=High  batteryTemperature=298.15 K  batteryTemperature_nominal_specify=off  batteryTemperature_nominal_value=1  batteryTemperature_nominal_unit=K  hysteresisState_specify=off  hysteresisState_priority=High  hysteresisState=0  hysteresisState_nominal_specify=off  hysteresisState_nominal_value=1  hysteresisState_nominal_unit=1  isExothermFaulted_specify=off  isExothermFaulted_priority=None  isExothermFaulted=0  isExothermFaulted_nominal_specify=off  isExothermFaulted_nominal_value=1  isExothermFaulted_nominal_unit=1  reactionHeatRate_specify=off  reactionHeatRate_priority=None  reactionHeatRate=0 W  reactionHeatRate_nominal_specify=off  reactionHeatRate_nominal_value=1  reactionHeatRate_nominal_unit=W  reactionExtent_specify=off  reactionExtent_priority=None  reactionExtent=0  reactionExtent_nominal_specify=off  reactionExtent_nominal_value=1  reactionExtent_nominal_unit=1
      settings: AttributesFormatString=Molicel:INR_21700_P45B
  Capacitor : ee_lib/Passive/Capacitor  cap_option=ee.enum.passive.capacitor.capOption.const  c=0.6 F  Cvec=[1e-05, 1e-06] F  Vvec=[0, 10] V  CV_table_symmetry=ee.enum.passive.capacitor.tableSymmetry.yes  f_vec=[1, 10] kHz  DFext_vec=[.8, 1.2]  enable_C_tol=ee.enum.toleranceApplication.none  averaging_period=0 s  C_tol=5  tol_distribution=ee.enum.toleranceDistribution.uniform  nSigma=4  r=0 Ohm  g=0 1/Ohm  enable_operating_limits=ee.enum.enable.no  operating_limit_action=ee.enum.passive.reportOpLim.warn  max_working_voltage_range=[-25, 25] V  power_rating=1 W  maxTemperature=85 degC  thermalEnable=false  thermalMass=1 J/K  i_specify=off  i_priority=None  i=0 A  i_nominal_specify=off  i_nominal_value=1  i_nominal_unit=A  v_specify=off  v_priority=None  v=40 V  v_nominal_specify=off  v_nominal_value=1  v_nominal_unit=V  vc_specify=off  vc_priority=High  vc=0 V  vc_nominal_specify=off  vc_nominal_value=1  vc_nominal_unit=V  T_specify=off  T_priority=None  T=298.15 K  T_nominal_specify=off  T_nominal_value=1  T_nominal_unit=K
  Constant1 : Constant  Value=50e-3
  Constant8 : Constant  Value=0
  Display : Display
  ERef Converter : fl_lib/Electrical/Electrical Elements/Electrical Reference
  Gate driver : Subsystem
  Inertia : fl_lib/Mechanical/Rotational Elements/Inertia  inertia="Jm  cm^2*g"  num_ports=foundation.enum.numPorts2.one  w_specify=on  w_priority=High  w=0 rpm  w_nominal_specify=off  w_nominal_value=1  w_nominal_unit=rad/s  t_specify=off  t_priority=High  t=0 N*m  t_nominal_specify=off  t_nominal_value=1  t_nominal_unit=N*m
  Inverter : ee_lib/Semiconductors & Converters/Converters/Converter (Three-Phase)  port_option=ee.enum.threePhasePort.composite  fidelity_option=ee.enum.converters.fidelity.detailed  device_type=ee.enum.converters.switchingdevice.igbt  showThermalPort=false  K=0  Vth=0.5 V  Vgt=1 V  Vgt_off=-1 V  Ih=1 A  Vf=0.8 V  Ron=0.001 Ohm  Rds=0.001 Ohm  Goff=1e-5 1/Ohm  Eon_scalar=22.86e-3 J  Eoff_scalar=17.14e-3 J  Eoff_natural_commutation=10e-3 J  Voff=300 V  Iout_scalar=600 A  onCurrentMeasDelay=0 s  useCurrentFromPreviousCycle=false  useVoltageFromPreviousCycle=false  diode_param=2  diode_Vf=0.8 V  diode_Ron=0.001 Ohm  diode_Goff=1e-5 1/Ohm  diode_C=50 nF  diode_iRM=-235 A  diode_iF=300 A  diode_idot=-50 A/us  diode_trr_param=1  diode_trr_factor=3  diode_trr=15 us  diode_Qrr=1.5e+3 s*uA  diode_rec_loss_model=ee.enum.diode.reverseRecoveryModel.fixed  diode_ErecVal=0 J  diode_scaleWithIandV=false  diode_ErecMat=zeros(2, 3) J  diode_TjrecVec=[298.15, 398.15] K  diode_IfrecVec=[.1, 1, 10] A  diode_IrecVal=10 A  diode_VrecVal=10 V  diode_tFilter=1 / 1000 / 100 s  thermal_network_parameterization=ee.enum.thermalNetworkTopology.external  Rth=[.08, .5] K/W  Rth_Cauer=[.08, .1, .5] K/W  Rth_Foster=[.08, .14, .22, .16] K/W  thermal_mass_parameterization=ee.enum.thermalNetwork.timeconstant  thermal_mass=[.01, .5] J/K  thermal_mass_Cauer=[.01, .1, .5] J/K  thermal_mass_Foster=[.001, .005, .05, .5] J/K  thermal_time_constant=[.001, .2] s  thermal_time_constant_Cauer=[.001, .1, .2] s  thermal_time_constant_Foster=[7e-05, .0007, .01, .08] s  thermal_mass_initial_temperatures=[25, 25] degC  thermal_mass_initial_temperatures_Cauer=[25, 25, 25] degC  junction_thermal_mass=0.01 J/K  Tvec_initial_Foster=[25, 25, 25, 25] degC  snubber_type=ee.enum.converters.snubber.exclude  Cs=1e-7 F  Rs=0.1 Ohm  Vce_loss=[0, 150, 300] V
  Is current calculation : Subsystem
  MRRef IPMSM : fl_lib/Mechanical/Rotational Elements/Mechanical Rotational Reference
  MRRef Load : fl_lib/Mechanical/Rotational Elements/Mechanical Rotational Reference
  Meas V : Subsystem
      mask Display: disp('Vdc')
  Rate Transition2 : RateTransition
  Rate Transition9 : RateTransition  OutPortSampleTime=Tsc
  Scope : Scope  NumInputPorts=2
      settings: ActiveDisplayYMinimum=-1  ActiveDisplayYMaximum=1  DataLoggingVariableName=ScopeData4
  Scope1 : Scope  NumInputPorts=2
      settings: ActiveDisplayYMinimum=-3.75  ActiveDisplayYMaximum=3.75  DataLoggingVariableName=ScopeData3
  Scope2 : Scope  NumInputPorts=2
      settings: ActiveDisplayYMinimum=-797.75076630434887  ActiveDisplayYMaximum=255.54428865855024  DataLoggingVariableName=ScopeData6
  Scopes : Subsystem
  Sensing trq : Subsystem
      mask Display: disp('trq')
  Sensing w a : Subsystem
      mask Display: disp('w,Hall')
  Sensing iabc : Subsystem
      mask Display: disp('iabc')
  Sign : Subsystem
  Simulink-PS Converter : nesl_utility/Simulink-PS Converter  PhysicalDomain=network_engine_domain  SubClassName=ps_input  LeftPortType=input  RightPortType=output  PseudoPeriodic=off  Frequencies=[]  NoiseDistribution=none  NoiseParameters=[]  Unit=N*m  AffineConversion=off  FilteringAndDerivatives=zero  SimscapeFilterOrder=1  InputFilterTimeConstant=0.001  UdotUserProvided=1
  Solver Configuration : nesl_utility/Solver Configuration  PhysicalDomain=network_engine_domain  SubClassName=solver  LeftPortType=input  RightPortType=generic  Tones=[]  Harmonics=[]  SimulateNoise=off  Profile=off  UseLocalSampling=off  EnableSwitchedLinearOptims=on  FrequencyDomain=off  UseCCode=off  RelTol=0.001  AbsTol=1e-06  MinStep=1e-09  ToWorkspace=off  RevertToSquareIcSolve=off  NumHomotopyIterations=100  PhasorMode=off  PhasorModeNumHarmonics=1  ConsistencySolver=NEWTON_FTOL  CanonicalOrdering=UNORDERED  OptimizeIntermediates=UNOPTIMIZED  IndexReductionMethod=DerivativeReplacement  DoDC=off  ResidualTolerance=1e-9  ConsistencyTolSource=GLOBAL  ConsistencyAbsTol=0.001  ConsistencyRelTol=0.001  ConsistencyTolFactor=0.001  UseLocalSolver=on  LocalSolverChoice=NE_TRAPEZOIDAL_ADVANCER  ResolveIndetEquations=on  FunctionEvalNumThread=1  LocalSolverSampleTime=Ts  DoFixedCost=on  MaxNonlinIter=4  MaxModeIter=2  ComputeImpulses=off  ImpulseIterations=2  LinearAlgebra=auto  LinearAlgebraNumThread=0  EquationFormulation=NE_TIME_EF  DelaysMemoryBudget=1024  AutomaticFiltering=on  FilteringTimeConstant=0.001  PartitionStorageMethod=AS_NEEDED  PartitionMemoryBudget=1024  PartitionMethod=FAST  MultibodyUseLocalSolver=off  MultibodyLocalSolverChoice=ODE1  MultibodyLocalSolverSampleTime=0.001
  Speed Controller : slpidlib/PID Controller  Controller=PI  Form=Parallel  TimeDomain=Discrete-time  UseExternalTs=off  SampleTime=-1  IntegratorMethod=Forward Euler  FilterMethod=Forward Euler  ControllerParametersSource=internal  P=0.003  I=2.1  UseKiTs=off  D=0.003  UseExternalDerivativeSource=off  N=100  UseFilter=on  TunerSelectOption=Transfer Function Based (PID Tuner App)  InitialConditionSource=internal  InitialConditionForIntegrator=0  InitialConditionForFilter=0  DifferentiatorICPrevScaledInput=0  ExternalReset=none  TrackingMode=off  Kt=1  LimitOutput=on  SatLimitsSource=internal  UpperSaturationLimit=3  LowerSaturationLimit=-3  LinearizeAsGain=on  AntiWindupMode=clamping  Kb=1  LimitIntegrator=on  UpperIntegratorSaturationLimit=3  LowerIntegratorSaturationLimit=-5  POutMin=[]  POutMax=[]  IOutMin=[]  IOutMax=[]  DOutMin=[]  DOutMax=[]  NOutMin=[]  NOutMax=[]  SumOutMin=[]  SumOutMax=[]  SaturationOutMin=[]  SaturationOutMax=[]  PParamMin=[]  PParamMax=[]  IParamMin=[]  IParamMax=[]  DParamMin=[]  DParamMax=[]  NParamMin=[]  NParamMax=[]  KbParamMin=[]  KbParamMax=[]  KtParamMin=[]  KtParamMax=[]  KbOutMin=[]  KbOutMax=[]  KtOutMin=[]  KtOutMax=[]  IntegratorOutMin=[]  IntegratorOutMax=[]  FilterOutMin=[]  FilterOutMax=[]  SumI1OutMin=[]  SumI1OutMax=[]  SumI2OutMin=[]  SumI2OutMax=[]  SumI3OutMin=[]  SumI3OutMax=[]  SumI4OutMin=[]  SumI4OutMax=[]  SumDOutMin=[]  SumDOutMax=[]  DifferentiatorOutMin=[]  DifferentiatorOutMax=[]  FilterDiffOutCoefMin=[]  FilterDiffOutCoefMax=[]  ReciprocalOutMin=[]  ReciprocalOutMax=[]  SumDenOutMin=[]  SumDenOutMax=[]  SumNumOutMin=[]  SumNumOutMax=[]  DivideOutMin=[]  DivideOutMax=[]  UdiffTsProdOutMin=[]  UdiffTsProdOutMax=[]  NTsProdOutMin=[]  NTsProdOutMax=[]  UintegralTsProdOutMin=[]  UintegralTsProdOutMax=[]  UngainTsProdOutMin=[]  UngainTsProdOutMax=[]  ClampingZeroOutDataTypeStr=Inherit: Inherit via back propagation  ClampingZeroOutMin=[]  ClampingZeroOutMax=[]  FilterDenConstantOutDataTypeStr=Inherit: Inherit via back propagation  FilterDenConstantOutMin=[]  FilterDenConstantOutMax=[]  PCopyOutDataTypeStr=Inherit: Inherit via back propagation  PCopyOutMin=[]  PCopyOutMax=[]  NCopyOutDataTypeStr=Inherit: Inherit via back propagation  NCopyOutMin=[]  NCopyOutMax=[]  IntegratorContinuousStateAttributes=''  IntegratorStateMustResolveToSignalObject=off  IntegratorRTWStateStorageClass=Auto  FilterContinuousStateAttributes=''  FilterStateMustResolveToSignalObject=off  FilterRTWStateStorageClass=Auto  ParallelPVariant=InternalParameters  IdealPVariant=Disabled  IVariant=InternalParameters  DVariant=Disabled  IntegratorVariant=Discrete  SatVariant=Enabled  AWVariant=DiscClampingParallel  PCopyVariant=Disabled  TRVariant=Disabled  FdbkBlocksVariant=Forward  IdealPFdbkVariant=Disabled  SatFdbkVariant=Disabled  DerivativeFilterVariant=Disabled  NVariant=Disabled  NCopyVariant=Disabled_SignalSpec  FilterICVariant=Disabled  IntegratorICVariant=InternalICs  ExternalResetVariant=Disabled  TRSumVariant=Passthrough  SumFdbkVariant=Disabled  SumVariant=Sum_PI  TsampFilterVariant=InternalTs  TsampNgainVariant=Passthrough  TsampIntegralVariant=Disabled_SignalSpec  ExternalSaturationOutDataTypeStr=Inherit: Same as second input  DerivativeSourceVariant=Disabled  PreIntVariant=InternalPreInt
  Sum : Sum  Inputs=|+-
  Torque Source : fl_lib/Mechanical/Mechanical Sources/Ideal Torque Source
  rpm output : Outport
  tag scope: dutcycle=global, load=global, rpm_ref=global
  wires:
  [iabc] -> Is current calculation/1(In1)
  Is current calculation/1(is) -> Scope/2, [is]
  Constant8/1 -> BLDC Current Controller with PWM Generation1/3
  Rate Transition2/1 -> Sum/2
  [Hall] -> Rate Transition9/1
  BLDC Current Controller with PWM Generation1/1 -> Gate driver/1(S), [dutcycle]
  Rate Transition9/1 -> BLDC Current Controller with PWM Generation1/4  "hall_signal"
  [is] -> Scope1/2, BLDC Current Controller with PWM Generation1/2  "is"
  rpm command/1 -> Sum/1, Sign/1(u), [rpm_ref], Display/1
  [load] -> Simulink-PS Converter/1
  Sum/1 -> Scope2/2, Speed Controller/1  "w_error"
  Constant1/1 -> [load]
  Speed Controller/1 -> Scope1/1, BLDC Current Controller with PWM Generation1/1, Scope2/1  "I_ref"
  [rpm] -> rpm output/1, Rate Transition2/1
  [dutcycle] -> Scope/1
  Sign/1(y) -> BLDC Current Controller with PWM Generation1/5  "direction"
  connections:
  Sensing iabc/RConn1 -- BLDC2/LConn1
  Torque Source/RConn1 -- Simulink-PS Converter/RConn1
  Meas V/LConn1 -- Battery Equivalent Circuit/LConn1 -- Capacitor/LConn1 -- Inverter/RConn1
  Gate driver/RConn1 -- Inverter/LConn1
  Sensing w a/LConn1 -- Torque Source/LConn1 -- Inertia/LConn1 -- Sensing trq/RConn1
  Solver Configuration/RConn1 -- MRRef Load/LConn1 -- Torque Source/RConn2
  Sensing trq/LConn1 -- BLDC2/RConn1
  Sensing iabc/LConn1 -- Inverter/LConn2
  BLDC2/RConn2 -- MRRef IPMSM/LConn1
  Meas V/RConn1 -- Battery Equivalent Circuit/RConn1 -- Capacitor/RConn1 -- ERef Converter/LConn1 -- Inverter/RConn2

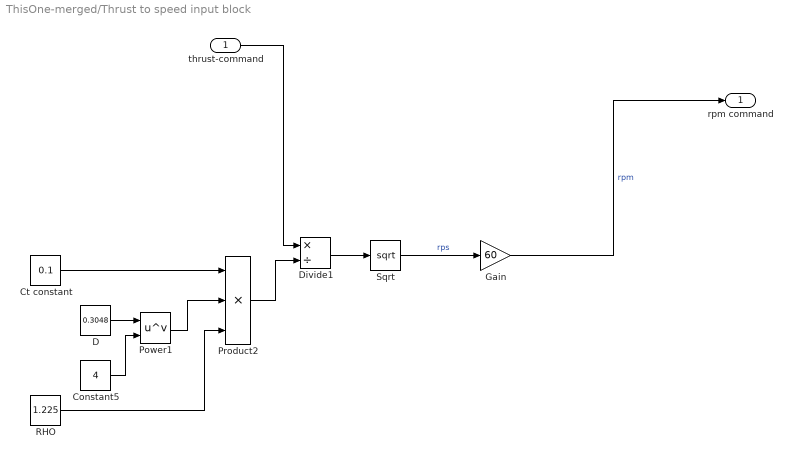
== system ThisOne-merged/Thrust to speed input block ==
  thrust-command : Inport
  Constant5 : Constant  Value=4
  Ct constant : Constant  Value=0.1
  D : Constant  Value=0.3048
  Divide1 : Product  Inputs=*/
  Gain : Gain  Gain=60
  Power1 : Math  Operator=pow
  Product2 : Product  Inputs=3
  RHO : Constant  Value=1.225
  Sqrt : Sqrt
  rpm command : Outport
  wires:
  Power1/1 -> Product2/2
  Constant5/1 -> Power1/2
  Sqrt/1 -> Gain/1  "rps"
  Ct constant/1 -> Product2/1
  RHO/1 -> Product2/3
  Divide1/1 -> Sqrt/1
  Gain/1 -> rpm command/1  "rpm"
  Product2/1 -> Divide1/2
  thrust-command/1 -> Divide1/1
  D/1 -> Power1/1
